simulink model "angle_control_model"  (R2019a)
settings: Solver=ode4  StartTime=0.0  StopTime=endtime  FixedStep=0.001  RelTol=1e-3
undefined symbols (not defined in the file or in its folder): Bd, K
settings Model: Creator=chris  LastModifiedBy=chris

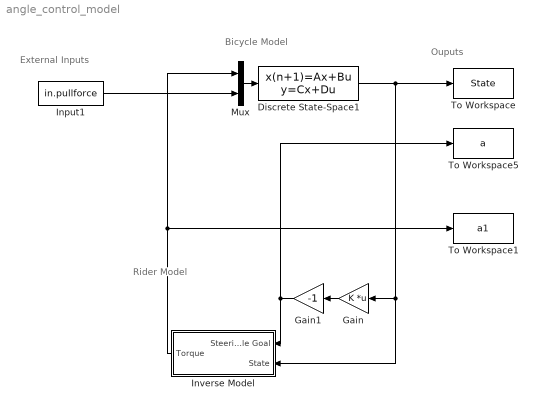
== system angle_control_model ==
  note: Bicycle Model
  note: External Inputs
  note: Rider Model
  note: Ouputs
  Discrete State-Space1 : DiscreteStateSpace  A=Bd.A  B=Bd.B  C=Bd.C  D=Bd.D  SampleTime=-1
  Gain : Gain  Gain=K  Multiplication=Matrix(K*u) (u vector)
  Gain1 : Gain  Gain=-1
  Input1 : FromWorkspace  VariableName=in.pullforce  SampleTime=0
  "Inverse Model " : Subsystem
  Mux : Mux  Inputs=2
  To Workspace : ToWorkspace  VariableName=State  SampleTime=-1
  To Workspace1 : ToWorkspace  VariableName=a1  SampleTime=-1
  To Workspace5 : ToWorkspace  VariableName=a  SampleTime=-1
  wires:
  Mux/1 -> Discrete State-Space1/1
  Input1/1 -> Mux/2
  Discrete State-Space1/1 -> "Inverse Model "/2("State "), Gain/1, To Workspace/1
  Gain/1 -> Gain1/1
  Gain1/1 -> To Workspace5/1, "Inverse Model "/1(Steering Angle Goal)
  "Inverse Model "/1(Torque) -> To Workspace1/1, Mux/1

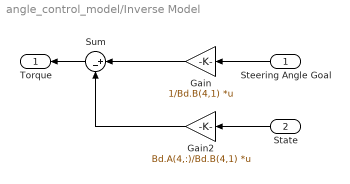
== system angle_control_model/Inverse Model  ==
  Steering Angle Goal : Inport
  "State " : Inport  Port=2
  Gain : Gain  Gain=1/Bd.B(4,1)  Multiplication=Matrix(K*u) (u vector)
  Gain2 : Gain  Gain=Bd.A(4,:)/Bd.B(4,1)  Multiplication=Matrix(K*u) (u vector)
  Sum : Sum  Inputs=|+-
  Torque : Outport
  wires:
  Steering Angle Goal/1 -> Gain/1
  Gain/1 -> Sum/1
  "State "/1 -> Gain2/1
  Gain2/1 -> Sum/2
  Sum/1 -> Torque/1
